simulink model "plant_model_for_linearization"  (R2015a)
settings: Solver=ode45  StartTime=0.0  StopTime=10.0  RelTol=1e-3
model workspace (MATLAB code in the model file):
  | %% Variables setup
  | m = 0.058; % [kg]
  | u_max = 12.28; % [V]
  | g = 9.81; % [m/s^2]
  | R_e = 4.38; % [Ohm]
  | % L(z) parameters: (L(z) - [mH], scaled in the model)
  | a = 27.62;
  | b = -304.84;
  | c = 112.75;
  | d = -2.74;
  | 
  | %% Initial conditions
  | z0 = 0.010; % [m]
  | z_min = 0;
  | z_max = 0.025; % [m]
  | i_min = 0;
  | v0 = 0.0; % [m/s]
  | 
  | sim_time = 1.5; % [s]
settings Model: Creator=Student  LastModifiedBy=Student
settings DataIOCC: LimitDataPoints=off

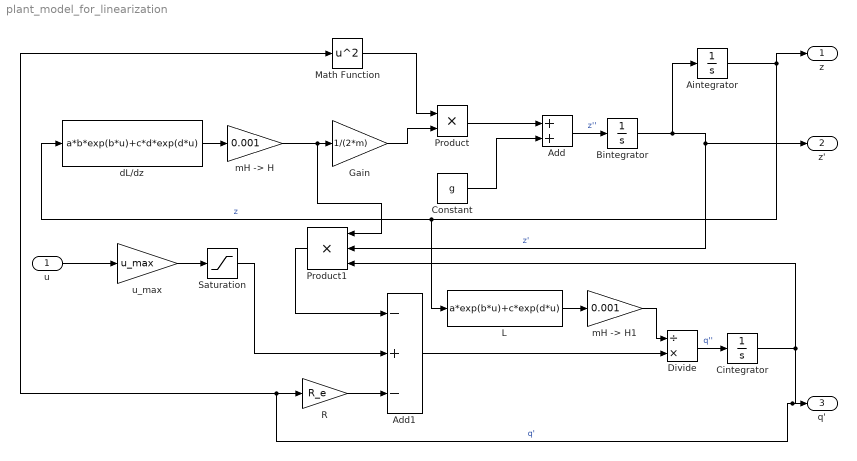
== system plant_model_for_linearization ==
  u : Inport
  Add : Sum
  Add1 : Sum  Inputs=-+-
  Aintegrator : Integrator  InitialCondition=z0  LimitOutput=on  UpperSaturationLimit=z_max  LowerSaturationLimit=z_min
  Bintegrator : Integrator
  Cintegrator : Integrator  LimitOutput=on  LowerSaturationLimit=i_min
  Constant : Constant  Value=g
  Divide : Product  Inputs=/*
  Gain : Gain  Gain=1/(2*m)
  L : Fcn  Expr=a*exp(b*u)+c*exp(d*u)
  Math Function : Math  Operator=square  SaturateOnIntegerOverflow=on
  Product : Product
  Product1 : Product  Inputs=3
  R : Gain  Gain=R_e
  Saturation : Saturate  UpperLimit=u_max  LowerLimit=0
  dL/dz : Fcn  Expr=a*b*exp(b*u)+c*d*exp(d*u)
  "mH -> H" : Gain  Gain=0.001
  "mH -> H1" : Gain  Gain=0.001
  u_max : Gain  Gain=u_max
  z : Outport
  z' : Outport  Port=2
  q' : Outport  Port=3
  wires:
  Math Function/1 -> Product/1
  Constant/1 -> Add/2
  Product/1 -> Add/1
  Gain/1 -> Product/2
  Bintegrator/1 -> Aintegrator/1, Product1/2, z'/1  "z'"
  R/1 -> Add1/3
  Add/1 -> Bintegrator/1  "z''"
  Saturation/1 -> Add1/2
  u/1 -> u_max/1
  u_max/1 -> Saturation/1
  Cintegrator/1 -> R/1, Math Function/1, q'/1, Product1/3  "q'"
  Divide/1 -> Cintegrator/1  "q''"
  Aintegrator/1 -> dL/dz/1, L/1, z/1  "z"
  Product1/1 -> Add1/1
  dL/dz/1 -> "mH -> H"/1
  Add1/1 -> Divide/2
  "mH -> H"/1 -> Product1/1, Gain/1
  L/1 -> "mH -> H1"/1
  "mH -> H1"/1 -> Divide/1
